simulink model "octave"  (R2018a)
settings: Solver=ode23t  StartTime=0.0  StopTime=3  MaxStep=1e-5  RelTol=1e-3
libraries: powerlib x15, dspvision x2, simulink x1, simulink_extras x1
settings Model: Creator=chris  LastModifiedBy=chris

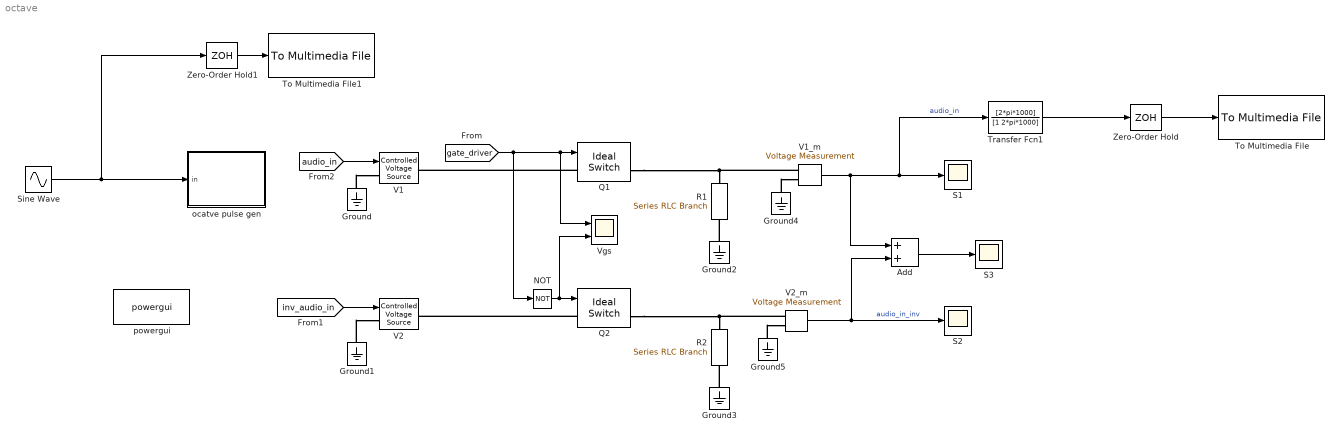
== system octave ==
  Add : Sum
  Ground{,1..5} (6 alike) : powerlib/Elements/Ground  LConnTagsString=a
  NOT : Logic  Operator=NOT  IconShape=distinctive  AllPortsSameDT=off  OutDataTypeStr=boolean
  Q1 : powerlib/Power Electronics/Ideal Switch  Ron=0.001  Lon=0  IC=0  Rs=1e5  Cs=inf  Measurements=on
  Q2 : powerlib/Power Electronics/Ideal Switch  Ron=0.001  Lon=0  IC=0  Rs=1e5  Cs=inf  Measurements=on
  R1 : powerlib/Elements/Series RLC Branch  LConnTagsString=__new0  RConnTagsString=__new0  BranchType=R  Resistance=10  Inductance=0  SetiL0=off  InitialCurrent=0  Capacitance=0  Setx0=off  InitialVoltage=0  Measurements=None
  R2 : powerlib/Elements/Series RLC Branch  LConnTagsString=__new0  RConnTagsString=__new0  BranchType=R  Resistance=10  Inductance=0  SetiL0=off  InitialCurrent=0  Capacitance=0  Setx0=off  InitialVoltage=0  Measurements=None
  S1 : Scope
  S2 : Scope
  S3 : Scope
  Sine Wave : Sin  Frequency=2*pi*440
  To Multimedia File : dspvision/To Multimedia File  outputFilename=octave.wav  streamSelection=Audio only  videoCompressor=None (uncompressed)  audioCompressor=None (uncompressed)  imagePorts=Separate color signals  fileType=WAV  audioDatatype=16-bit integer  fourcc=RGB  videoQuality=75  mj2000CompFactor=10
      settings: SourceProductName=Computer Vision System Toolbox  SourceProductBaseCode=VP
  To Multimedia File1 : dspvision/To Multimedia File  outputFilename=original.wav  streamSelection=Audio only  videoCompressor=None (uncompressed)  audioCompressor=None (uncompressed)  imagePorts=Separate color signals  fileType=WAV  audioDatatype=16-bit integer  fourcc=RGB  videoQuality=75  mj2000CompFactor=10
      settings: SourceProductName=Computer Vision System Toolbox  SourceProductBaseCode=VP
  Transfer Fcn1 : TransferFcn  InitFcn=fc=300,  Numerator=[2*pi*1000]  Denominator=[1 2*pi*1000]
  V1 : powerlib/Electrical Sources/Controlled Voltage Source  Initialize=on  Source_Type=AC  Amplitude=0  Phase=0  Frequency=0  Measurements=None
  V1_m : powerlib/Measurements/Voltage Measurement  PhasorSimulation=off  OutputType=Complex  PSBequivalent=0
  V2 : powerlib/Electrical Sources/Controlled Voltage Source  Initialize=on  Source_Type=AC  Amplitude=0  Phase=0  Frequency=0  Measurements=None
  V2_m : powerlib/Measurements/Voltage Measurement  PhasorSimulation=off  OutputType=Complex  PSBequivalent=0
  Vgs : Scope  NumInputPorts=2
  Zero-Order Hold : ZeroOrderHold  SampleTime=-1
  Zero-Order Hold1 : ZeroOrderHold  SampleTime=-1
  ocatve pulse gen : Subsystem
  powergui : powerlib/powergui  Priority=1  SimulationMode=Continuous  SampleTime=50e-6  frequency=60  Iterations=50  frequencyindice=0  Pbase=100e6  ErrMax=1e-4  UnitsV=kV  UnitsW=MW  buscounter=0  FunctionMessages=off  echomessages=off  EnableUseOfTLC=off  CurrentSourceSwitches=off  DisableSnubberDevices=off  DisableRonSwitches=on  DisableVfSwitches=on  DisplayEquations=off  SolverType=Tustin/Backward Euler (TBE)  Interpol=off  ExternalGateDelay=off  methode=off  Ts=100  x0status=blocks  SPID=on  SwTol=0  HookPort=off  RestoreLinks=warning  ResistiveCurrentMeasurement=off  Frange=[0:2:500]  Ylog=off  Xlog=on  ShowGrid=off  save=off  variable=ZData  structure=0  ZoomFFT=off  StartTime=0.0  cycles=1  DisplayStyle=1  fundamental=60  FreqAxis=off  MaxFrequency=1000  frequencyindicesteady=1  RmsSteady=1  display=off
  wires:
  Zero-Order Hold/1 -> To Multimedia File/1
  [audio_in] -> V1/1
  [inv_audio_in] -> V2/1
  V1_m/1 -> Add/1, Transfer Fcn1/1, S1/1  "audio_in"
  V2_m/1 -> Add/2, S2/1  "audio_in_inv"
  [gate_driver] -> Q1/1, Vgs/1, NOT/1
  NOT/1 -> Q2/1, Vgs/2
  Sine Wave/1 -> Zero-Order Hold1/1, ocatve pulse gen/1(in)
  Zero-Order Hold1/1 -> To Multimedia File1/1
  Transfer Fcn1/1 -> Zero-Order Hold/1
  Add/1 -> S3/1
  connections:
  Ground2/LConn1 -- R1/RConn1
  Ground/LConn1 -- V1/LConn1
  Ground1/LConn1 -- V2/LConn1
  Q1/LConn1 -- V1/RConn1
  Q2/LConn1 -- V2/RConn1
  Ground3/LConn1 -- R2/RConn1
  R1/LConn1 -- Q1/RConn1 -- V1_m/LConn1
  R2/LConn1 -- Q2/RConn1 -- V2_m/LConn1
  Ground4/LConn1 -- V1_m/LConn2
  Ground5/LConn1 -- V2_m/LConn2

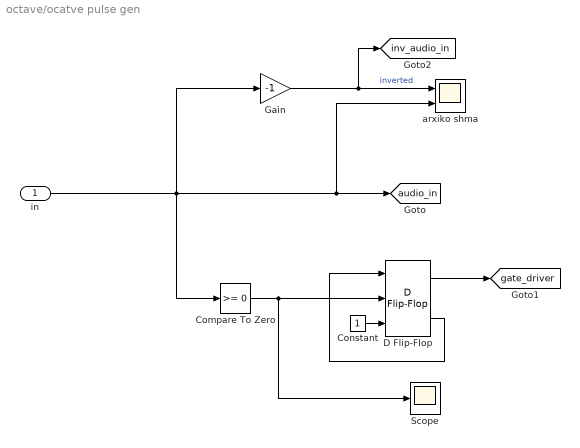
== system octave/ocatve pulse gen ==
  in : Inport
  Compare To Zero : simulink/Logic and Bit Operations/Compare To Zero  relop=>=  OutDataTypeStr=boolean
  Constant : Constant  OutDataTypeStr=boolean
  D Flip-Flop : simulink_extras/Flip Flops/D Flip-Flop
      settings: SourceProductName=Simulink
  Gain : Gain  Gain=-1
  Scope : Scope
  arxiko shma : Scope  NumInputPorts=2
  tag scope: audio_in=global, gate_driver=global, inv_audio_in=global
  wires:
  in/1 -> Gain/1, Compare To Zero/1, arxiko shma/2, [audio_in]
  Constant/1 -> D Flip-Flop/3
  D Flip-Flop/1 -> [gate_driver]
  D Flip-Flop/2 -> D Flip-Flop/1
  Gain/1 -> [inv_audio_in], arxiko shma/1  "inverted"
  Compare To Zero/1 -> D Flip-Flop/2, Scope/1
